simulink model "Buck_Converter_Plant_Model"  (R2021a)
settings: Solver=ode15s  StartTime=0.0  StopTime=2  RelTol=1e-3
values from neighbouring files (symbols this model uses):
  Cx = 100e-6    (= 0.0001)    [Buck_Converter_Simulation.m]
  f_err = 20    [Buck_Converter_Simulation.m]
  f_sw = 20e3    (= 20000)    [Buck_Converter_Simulation.m]
  L = 400e-6    (= 0.0004)    [Buck_Converter_Simulation.m]
  Rerr = 0.15    [Buck_Converter_Simulation.m]
  Ro = 50    [Buck_Converter_Simulation.m]
  Verr = 0.05    [Buck_Converter_Simulation.m]
  Vin = 400    [Buck_Converter_Simulation.m]
libraries: eePwmGenerator x1
settings Model: Creator=byuwono2022  LastModifiedBy=byuwono2022

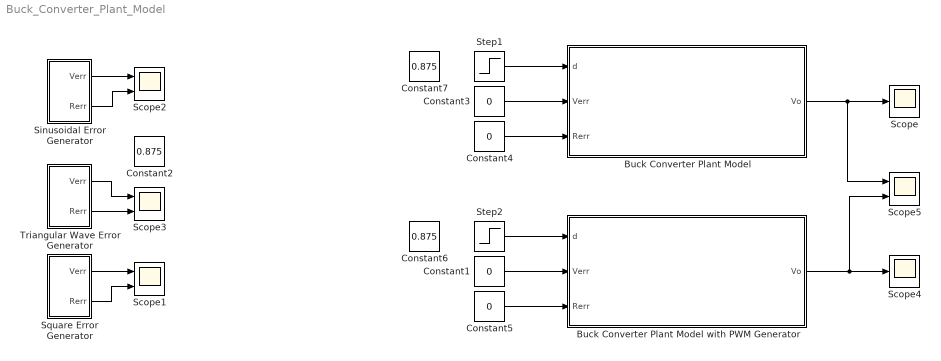
== system Buck_Converter_Plant_Model ==
  Buck Converter Plant Model : Subsystem
  Buck Converter Plant Model with PWM Generator : Subsystem
  Constant{1,3..5} (4 alike) : Constant  Value=0
  Constant2 : Constant  Value=0.875
  Constant6 : Constant  Value=0.875
  Constant7 : Constant  Value=0.875
  Scope : Scope
  Scope{1..3,5} (4 alike) : Scope  NumInputPorts=2
  Scope4 : Scope
  Sinusoidal Error Generator : Subsystem
  Square Error Generator : Subsystem
  Step1 : Step  After=0.875  SampleTime=0
  Step2 : Step  After=0.875  SampleTime=0
  Triangular Wave Error Generator : Subsystem
  wires:
  Buck Converter Plant Model/1(Vo) -> Scope5/1, Scope/1
  Square Error Generator/1(Verr) -> Scope1/1
  Square Error Generator/2(Rerr) -> Scope1/2
  Constant3/1 -> Buck Converter Plant Model/2(Verr)
  Constant4/1 -> Buck Converter Plant Model/3(Rerr)
  Sinusoidal Error Generator/1(Verr) -> Scope2/1
  Sinusoidal Error Generator/2(Rerr) -> Scope2/2
  Triangular Wave Error Generator/1(Verr) -> Scope3/1
  Triangular Wave Error Generator/2(Rerr) -> Scope3/2
  Step1/1 -> Buck Converter Plant Model/1(d)
  Constant5/1 -> Buck Converter Plant Model with PWM Generator/3(Rerr)
  Constant1/1 -> Buck Converter Plant Model with PWM Generator/2(Verr)
  Buck Converter Plant Model with PWM Generator/1(Vo) -> Scope5/2, Scope4/1
  Step2/1 -> Buck Converter Plant Model with PWM Generator/1(d)

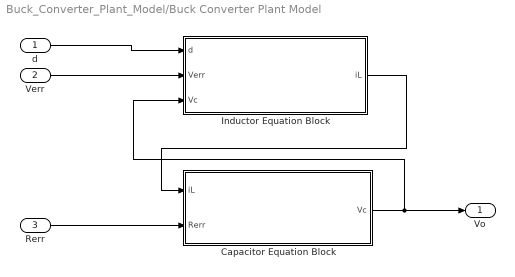
== system Buck_Converter_Plant_Model/Buck Converter Plant Model ==
  d : Inport
  Verr : Inport  Port=2
  Rerr : Inport  Port=3
  Capacitor Equation Block : Subsystem
  Inductor Equation Block : Subsystem
  Vo : Outport
  wires:
  Inductor Equation Block/1(iL) -> Capacitor Equation Block/1(iL)
  Capacitor Equation Block/1(Vc) -> Vo/1, Inductor Equation Block/3(Vc)
  Verr/1 -> Inductor Equation Block/2(Verr)
  Rerr/1 -> Capacitor Equation Block/2(Rerr)
  d/1 -> Inductor Equation Block/1(d)

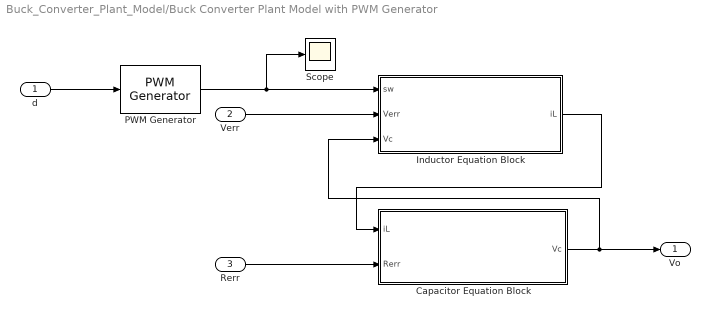
== system Buck_Converter_Plant_Model/Buck Converter Plant Model with PWM Generator ==
  d : Inport
  Verr : Inport  Port=2
  Rerr : Inport  Port=3
  Capacitor Equation Block : Subsystem
  Inductor Equation Block : Subsystem
  PWM Generator : eePwmGenerator/PWM Generator  CarrCount=Up  Tper=1/f_sw  Ts=0
  Scope : Scope
  Vo : Outport
  wires:
  Inductor Equation Block/1(iL) -> Capacitor Equation Block/1(iL)
  Capacitor Equation Block/1(Vc) -> Vo/1, Inductor Equation Block/3(Vc)
  Verr/1 -> Inductor Equation Block/2(Verr)
  Rerr/1 -> Capacitor Equation Block/2(Rerr)
  PWM Generator/1 -> Scope/1, Inductor Equation Block/1(sw)
  d/1 -> PWM Generator/1

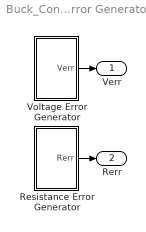
== system Buck_Converter_Plant_Model/Sinusoidal Error Generator ==
  Resistance Error Generator : Subsystem
  Voltage Error Generator : Subsystem
  Verr : Outport
  Rerr : Outport  Port=2
  wires:
  Voltage Error Generator/1(Verr) -> Verr/1
  Resistance Error Generator/1(Rerr) -> Rerr/1

== system Buck_Converter_Plant_Model/Square Error Generator ==
  Resistance Error Generator : Subsystem
  Voltage Error Generator : Subsystem
  Verr : Outport
  Rerr : Outport  Port=2
  wires:
  Voltage Error Generator/1(Verr) -> Verr/1
  Resistance Error Generator/1(Rerr) -> Rerr/1

== system Buck_Converter_Plant_Model/Triangular Wave Error Generator ==
  Resistance Error Generator : Subsystem
  Voltage Error Generator : Subsystem
  Verr : Outport
  Rerr : Outport  Port=2
  wires:
  Voltage Error Generator/1(Verr) -> Verr/1
  Resistance Error Generator/1(Rerr) -> Rerr/1

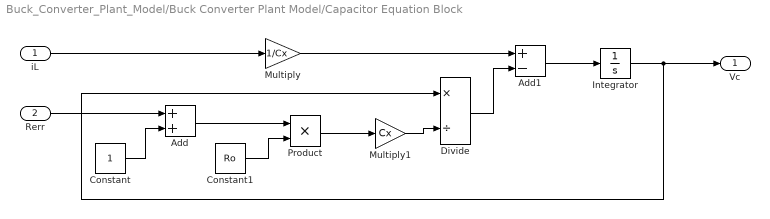
== system Buck_Converter_Plant_Model/Buck Converter Plant Model/Capacitor Equation Block ==
  iL : Inport
  Rerr : Inport  Port=2
  Add : Sum
  Add1 : Sum  Inputs=+-
  Constant : Constant
  Constant1 : Constant  Value=Ro
  Divide : Product  Inputs=*/
  Integrator : Integrator  InitialCondition=0.0000000001
  Multiply : Gain  Gain=1/Cx
  Multiply1 : Gain  Gain=Cx
  Product : Product
  Vc : Outport
  wires:
  Integrator/1 -> Vc/1, Divide/1
  iL/1 -> Multiply/1
  Multiply1/1 -> Divide/2
  Constant/1 -> Add/2
  Rerr/1 -> Add/1
  Add1/1 -> Integrator/1
  Add/1 -> Product/1
  Constant1/1 -> Product/2
  Product/1 -> Multiply1/1
  Divide/1 -> Add1/2
  Multiply/1 -> Add1/1

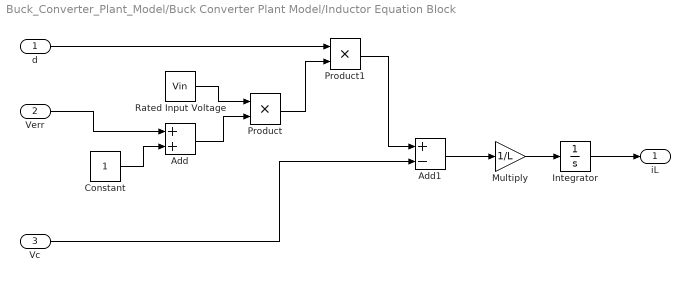
== system Buck_Converter_Plant_Model/Buck Converter Plant Model/Inductor Equation Block ==
  d : Inport
  Verr : Inport  Port=2
  Vc : Inport  Port=3
  Add : Sum
  Add1 : Sum  Inputs=+-
  Constant : Constant
  Integrator : Integrator  InitialCondition=0.0000000001
  Multiply : Gain  Gain=1/L
  Product : Product
  Product1 : Product
  Rated Input Voltage : Constant  Value=Vin
  iL : Outport
  wires:
  Multiply/1 -> Integrator/1
  Vc/1 -> Add1/2
  Product/1 -> Product1/2
  Add/1 -> Product/2
  Integrator/1 -> iL/1
  Verr/1 -> Add/1
  Product1/1 -> Add1/1
  d/1 -> Product1/1
  Add1/1 -> Multiply/1
  Constant/1 -> Add/2
  Rated Input Voltage/1 -> Product/1

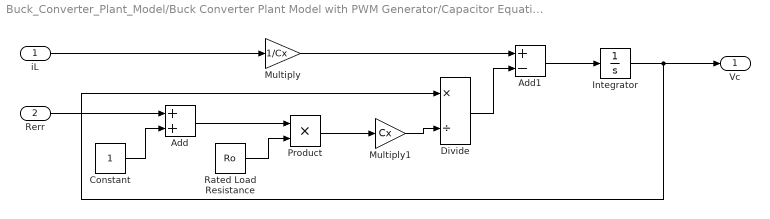
== system Buck_Converter_Plant_Model/Buck Converter Plant Model with PWM Generator/Capacitor Equation Block ==
  iL : Inport
  Rerr : Inport  Port=2
  Add : Sum
  Add1 : Sum  Inputs=+-
  Constant : Constant
  Divide : Product  Inputs=*/
  Integrator : Integrator
  Multiply : Gain  Gain=1/Cx
  Multiply1 : Gain  Gain=Cx
  Product : Product
  Rated Load Resistance : Constant  Value=Ro
  Vc : Outport
  wires:
  Integrator/1 -> Vc/1, Divide/1
  iL/1 -> Multiply/1
  Multiply1/1 -> Divide/2
  Constant/1 -> Add/2
  Rerr/1 -> Add/1
  Add1/1 -> Integrator/1
  Add/1 -> Product/1
  Rated Load Resistance/1 -> Product/2
  Product/1 -> Multiply1/1
  Divide/1 -> Add1/2
  Multiply/1 -> Add1/1

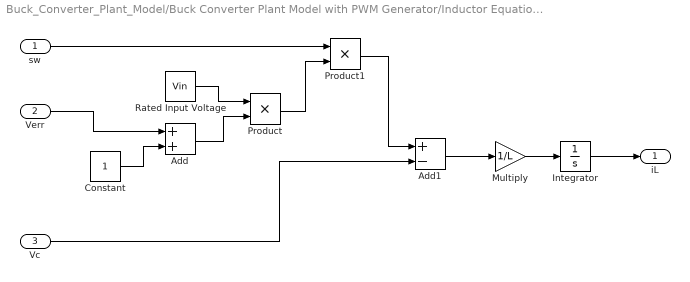
== system Buck_Converter_Plant_Model/Buck Converter Plant Model with PWM Generator/Inductor Equation Block ==
  sw : Inport
  Verr : Inport  Port=2
  Vc : Inport  Port=3
  Add : Sum
  Add1 : Sum  Inputs=+-
  Constant : Constant
  Integrator : Integrator
  Multiply : Gain  Gain=1/L
  Product : Product
  Product1 : Product
  Rated Input Voltage : Constant  Value=Vin
  iL : Outport
  wires:
  Multiply/1 -> Integrator/1
  Vc/1 -> Add1/2
  Product/1 -> Product1/2
  Add/1 -> Product/2
  Integrator/1 -> iL/1
  Verr/1 -> Add/1
  Product1/1 -> Add1/1
  sw/1 -> Product1/1
  Add1/1 -> Multiply/1
  Constant/1 -> Add/2
  Rated Input Voltage/1 -> Product/1

== system Buck_Converter_Plant_Model/Sinusoidal Error Generator/Resistance Error Generator ==
  Product : Product
  Signal Generator : SignalGenerator  Amplitude=Rerr  Frequency=f_err
  Step2 : Step  Time=6  SampleTime=0
  Rerr : Outport
  wires:
  Signal Generator/1 -> Product/1
  Step2/1 -> Product/2
  Product/1 -> Rerr/1

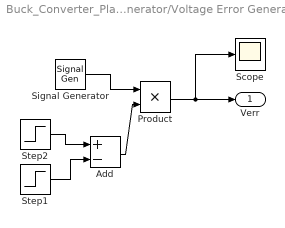
== system Buck_Converter_Plant_Model/Sinusoidal Error Generator/Voltage Error Generator ==
  Add : Sum  Inputs=+-
  Product : Product
  Scope : Scope
  Signal Generator : SignalGenerator  Amplitude=Verr  Frequency=f_err
  Step1 : Step  Before=1  After=0  SampleTime=0
  Step2 : Step  Time=5  Before=1  After=0  SampleTime=0
  Verr : Outport
  wires:
  Signal Generator/1 -> Product/1
  Product/1 -> Scope/1, Verr/1
  Add/1 -> Product/2
  Step2/1 -> Add/1
  Step1/1 -> Add/2

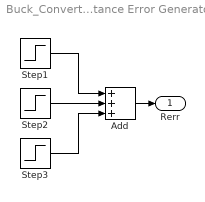
== system Buck_Converter_Plant_Model/Square Error Generator/Resistance Error Generator ==
  Add : Sum  Inputs=+++
  Step1 : Step  Time=5.5  After=Rerr  SampleTime=0
  Step2 : Step  Time=6.5  After=-2*Rerr  SampleTime=0
  Step3 : Step  Time=7.5  After=Rerr  SampleTime=0
  Rerr : Outport
  wires:
  Step3/1 -> Add/3
  Step2/1 -> Add/2
  Step1/1 -> Add/1
  Add/1 -> Rerr/1

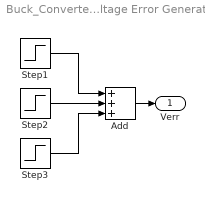
== system Buck_Converter_Plant_Model/Square Error Generator/Voltage Error Generator ==
  Add : Sum  Inputs=+++
  Step1 : Step  Time=2  After=Verr  SampleTime=0
  Step2 : Step  Time=3  After=-2*Verr  SampleTime=0
  Step3 : Step  Time=4  After=Verr  SampleTime=0
  Verr : Outport
  wires:
  Step3/1 -> Add/3
  Step2/1 -> Add/2
  Step1/1 -> Add/1
  Add/1 -> Verr/1

== system Buck_Converter_Plant_Model/Triangular Wave Error Generator/Resistance Error Generator ==
  Product : Product
  Signal Generator : SignalGenerator  WaveForm=sawtooth  Amplitude=Rerr  Frequency=f_err
  Step2 : Step  Time=6  SampleTime=0
  Rerr : Outport
  wires:
  Signal Generator/1 -> Product/1
  Step2/1 -> Product/2
  Product/1 -> Rerr/1

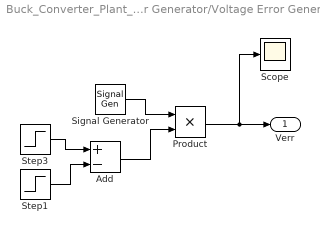
== system Buck_Converter_Plant_Model/Triangular Wave Error Generator/Voltage Error Generator ==
  Add : Sum  Inputs=+-
  Product : Product
  Scope : Scope
  Signal Generator : SignalGenerator  WaveForm=sawtooth  Amplitude=Verr  Frequency=f_err
  Step1 : Step  Before=1  After=0  SampleTime=0
  Step3 : Step  Time=5  Before=1  After=0  SampleTime=0
  Verr : Outport
  wires:
  Signal Generator/1 -> Product/1
  Add/1 -> Product/2
  Product/1 -> Scope/1, Verr/1
  Step3/1 -> Add/1
  Step1/1 -> Add/2
